simulink model "model_affc"  (R2016b)
settings: Solver=FixedStepDiscrete  StartTime=0.0  StopTime=inf  FixedStep=sampleTime  RelTol=1e-3
InitFcn:
  | model_affc_parameters;
StartFcn:
  | model_affc_parameters;
values from neighbouring files (symbols this model uses):
  Lb = 0.07    [model_affc_parameters.m]
  Lf = 0.238    [model_affc_parameters.m]
  Lu = 0.153    [model_affc_parameters.m]
  sampleTime = 0.001    [model_affc_parameters.m]
undefined symbols (not defined in the file or in its folder): FM1
libraries: simulink x11, LibraryFM x10, VariousBlocksLibrary x2, FMLibrary_v2 x1
settings Model: SimulationMode=external  Creator=niekbeckers  LastModifiedBy=Labuser
settings DataIOCC: LimitDataPoints=on  SaveFormat=Array
settings OptimizationCC: BlockReduction=off  BooleanDataType=off  LocalBlockOutputs=off  LifeSpan=inf
settings DebuggingCC: SaveWithParameterizedLinksMsg=none  UnderspecifiedInitializationDetection=Classic  MergeDetectMultiDrivingBlocksExec=none  SignalResolutionControl=TryResolveAllWithWarning  SFUnexpectedBacktrackingDiag=warning  SFNoUnconditionalDefaultTransitionDiag=warning  SFExecutionAtInitializationDiag=none
settings HardwareCC: ProdBitPerPointer=32  ProdBitPerSizeT=32  ProdBitPerPtrDiffT=32  ProdLargestAtomicFloat=None  ProdIntDivRoundTo=Undefined  ProdEndianess=Unspecified  ProdWordSize=32  ProdHWDeviceType=32-bit Generic  TargetBitPerPointer=64  TargetBitPerSizeT=64  TargetBitPerPtrDiffT=64  TargetLongLongMode=on  TargetIntDivRoundTo=Zero  TargetEndianess=LittleEndian  TargetWordSize=64  TargetHWDeviceType=MATLAB Host  ProdEqTarget=off
settings ModelReferenceCC: PropagateSignalLabelsOutOfModel=off
settings RTWCC: SystemTargetFile=TwinCAT.tlc  GenCodeOnly=on  MakeCommand=make_tct  TemplateMakefile=tct_msbuild.tmf  Description=TwinCAT Target  GenerateReport=on  TargetLang=C++
settings STFCustomTargetCC: CompOptLevelCompliant=on  GeneratePreprocessorConditionals=Disable all  MATLABClassNameForMDSCustomization=Simulink.SoftwareTarget.TargetSpecificTriggerConfigurationBase  SystemTargetFile=TwinCAT.tlc
settings ConfigComp: CovMetricSettings=dw  CovHtmlReporting=on  CovSaveCumulativeToWorkspaceVar=on  CovSaveSingleToWorkspaceVar=on  CovExternalEMLEnable=off  CovSFcnEnable=off

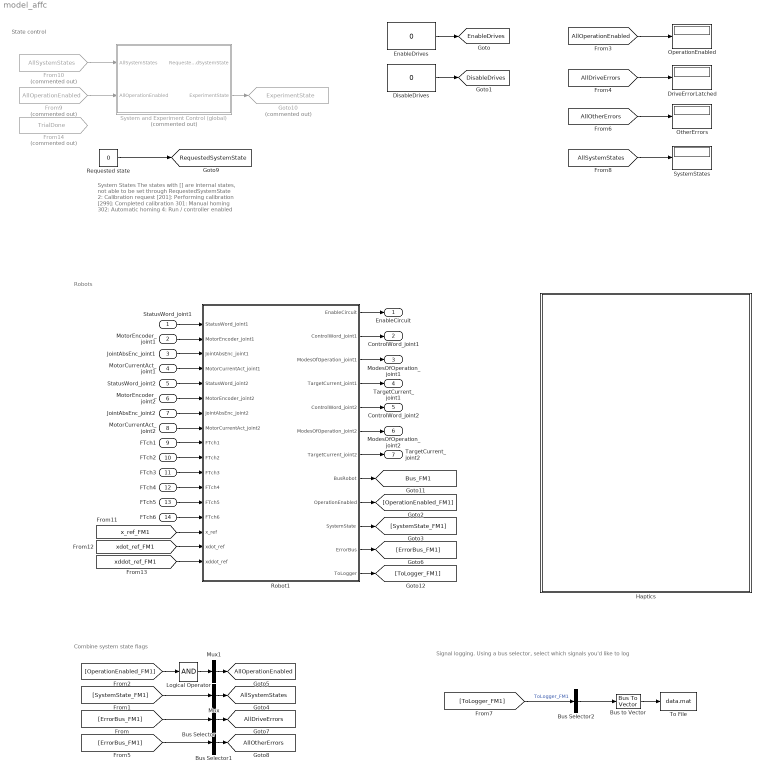
== system model_affc ==
  note: Signal logging.
      | Using a bus selector, select which signals you'd like to log
  note: System States
      | The states with [] are internal states, not able to be set through RequestedSystemState
      | 2: Calibration request
      | [201]: Performing calibration
      | [299]: Completed calibration
      | 301: Manual homing
      | 302: Automatic homing
      | 4: Run / controller enabled
  note: State control
  note: Combine system state flags
  note: Robots
  StatusWord_joint1 : Inport  OutDataTypeStr=uint16  PortDimensions=1
  MotorEncoder_joint1 : Inport  Port=2  OutDataTypeStr=int32  PortDimensions=1
  JointAbsEnc_joint1 : Inport  Port=3  OutDataTypeStr=int32  PortDimensions=1
  MotorCurrentAct_joint1 : Inport  Port=4  OutDataTypeStr=int16  PortDimensions=1
  StatusWord_joint2 : Inport  Port=5  OutDataTypeStr=uint16  PortDimensions=1
  MotorEncoder_joint2 : Inport  Port=6  OutDataTypeStr=int32  PortDimensions=1
  JointAbsEnc_joint2 : Inport  Port=7  OutDataTypeStr=int32  PortDimensions=1
  MotorCurrentAct_joint2 : Inport  Port=8  OutDataTypeStr=int16  PortDimensions=1
  FTch1 : Inport  Port=9  OutDataTypeStr=single  PortDimensions=1
  FTch2 : Inport  Port=10  OutDataTypeStr=single  PortDimensions=1
  FTch3 : Inport  Port=11  OutDataTypeStr=single  PortDimensions=1
  FTch4 : Inport  Port=12  OutDataTypeStr=single  PortDimensions=1
  FTch5 : Inport  Port=13  OutDataTypeStr=single  PortDimensions=1
  FTch6 : Inport  Port=14  OutDataTypeStr=single  PortDimensions=1
  Bus Selector : BusSelector  OutputSignals=DriveErrorLatched  OutputAsBus=on
  Bus Selector1 : BusSelector  OutputSignals=WorkspaceErrorLatched,ForceSensorLatched  OutputAsBus=on
  Bus Selector2 : BusSelector  OutputSignals=SystemState,ToLogger_ToEtherCAT.ToLogger_Actuator1.JointPosition_rad,ToLogger_ToEtherCAT.ToLogger_Actuator1.JointVelocity_rads,ToLogger_ToEtherCAT.ToLogger_Actuator1.JointTorque_Act_Nm,ToLogger_ToEtherCAT.ToLogger_Actuator1.DesiredTorqueLimited_Nm,ToLogger_ToEtherCAT.ToLogger_Actuator1.DriveError,ToLogger_ToEtherCAT.ToLogger_Actuator2.JointPosition_rad,ToLogger_ToEtherCAT.ToLogger_Actuator2.JointVelocity_rads,ToLogger_ToEtherCAT.ToLogger_Actuator2.JointTorque_Act_Nm,ToLogger_ToEtherCAT.ToLogger_Actuator2.DesiredTorqueLimited_Nm,ToLogger_ToEtherCAT.ToLogger_Actuator2.DriveError,ToLogger_Controller.q_ref,ToLogger_Controller.qdot_ref,ToLogger_Controller.qddot_ref  OutputAsBus=on
  Bus to Vector : BusToVector
  DisableDrives : Constant  Value=0
      settings: OpenFcn=set_param(gcb,'Value','1');tname = ['toggletimer_' gcb];delete(timerfind('name',tname));t = timer('timerfcn', ['set_param(''',gcb,''',''Value'',''0'')'],'executionmode','singleshot','startdelay',1,'name',tname);start(t);
      mask Display: fprintf('PushToTrigger\n%s',get_param(gcb,'value'))
  DriveErrorLatched : Display
  EnableDrives : Constant  Value=0
      settings: OpenFcn=set_param(gcb,'Value','1');tname = ['toggletimer_' gcb];delete(timerfind('name',tname));t = timer('timerfcn', ['set_param(''',gcb,''',''Value'',''0'')'],'executionmode','singleshot','startdelay',1,'name',tname);start(t);
      mask Display: fprintf('PushToTrigger\n%s',get_param(gcb,'value'))
  From10 : From  Commented=on  GotoTag=AllSystemStates
  From14 : From  Commented=on  GotoTag=TrialDone
  From9 : From  Commented=on  GotoTag=AllOperationEnabled
  Goto10 : Goto  Commented=on  GotoTag=ExperimentState  TagVisibility=global
  Haptics : Subsystem
  Logical Operator : Logic  Inputs=1  AllPortsSameDT=off  OutDataTypeStr=boolean
  Mux : Mux  Inputs=1
  Mux1 : Mux  Inputs=1
  OperationEnabled : Display
  OtherErrors : Display
  Requested state : Constant  Value=0
  Robot1 : Subsystem  AncestorBlock=LibraryFM/Robot1  mask{RobotStruct=FM1}
      mask prompts: RobotStruct "Robot struct (data)"
  System and Experiment Control (global) : Subsystem  Commented=on
  SystemStates : Display
  To File : ToFile  Filename=data.mat
  EnableCircuit : Outport  OutDataTypeStr=boolean  PortDimensions=1
  ControlWord_joint1 : Outport  Port=2  OutDataTypeStr=uint16  PortDimensions=1
  ModesOfOperation_joint1 : Outport  Port=3  OutDataTypeStr=int8  PortDimensions=1
  TargetCurrent_joint1 : Outport  Port=4  OutDataTypeStr=int16  PortDimensions=1
  ControlWord_joint2 : Outport  Port=5  OutDataTypeStr=uint16  PortDimensions=1
  ModesOfOperation_joint2 : Outport  Port=6  OutDataTypeStr=int8  PortDimensions=1
  TargetCurrent_joint2 : Outport  Port=7  OutDataTypeStr=int16  PortDimensions=1
  tag scope: AllDriveErrors=global, AllOperationEnabled=global, AllOtherErrors=global, AllSystemStates=global, Bus_FM1=global, DisableDrives=global, EnableDrives=global, RequestedSystemState=global
  wires:
  DisableDrives/1 -> [DisableDrives]
  EnableDrives/1 -> [EnableDrives]
  Robot1/9(OperationEnabled) -> [OperationEnabled_FM1]
  [AllOperationEnabled] -> OperationEnabled/1
  Robot1/10(SystemState) -> [SystemState_FM1]
  [SystemState_FM1] -> Mux/1
  Mux/1 -> [AllSystemStates]
  Mux1/1 -> [AllOperationEnabled]
  [OperationEnabled_FM1] -> Logical Operator/1
  Robot1/11(ErrorBus) -> [ErrorBus_FM1]
  [ErrorBus_FM1] -> Bus Selector/1
  Bus Selector/1 -> [AllDriveErrors]
  [AllDriveErrors] -> DriveErrorLatched/1
  [ErrorBus_FM1] -> Bus Selector1/1
  Bus Selector1/1 -> [AllOtherErrors]
  [AllOtherErrors] -> OtherErrors/1
  [AllSystemStates] -> SystemStates/1
  System and Experiment Control (global)/2(ExperimentState) -> Goto10/1
  From10/1 -> System and Experiment Control (global)/1(AllSystemStates)
  From9/1 -> System and Experiment Control (global)/2(AllOperationEnabled)
  [x_ref_FM1] -> Robot1/15(x_ref)
  [xdot_ref_FM1] -> Robot1/16(xdot_ref)
  [xddot_ref_FM1] -> Robot1/17(xddot_ref)
  Requested state/1 -> [RequestedSystemState]
  Robot1/8(BusRobot) -> [Bus_FM1]
  StatusWord_joint1/1 -> Robot1/1(StatusWord_joint1)
  MotorEncoder_joint1/1 -> Robot1/2(MotorEncoder_joint1)
  JointAbsEnc_joint1/1 -> Robot1/3(JointAbsEnc_joint1)
  MotorCurrentAct_joint1/1 -> Robot1/4(MotorCurrentAct_joint1)
  StatusWord_joint2/1 -> Robot1/5(StatusWord_joint2)
  MotorEncoder_joint2/1 -> Robot1/6(MotorEncoder_joint2)
  JointAbsEnc_joint2/1 -> Robot1/7(JointAbsEnc_joint2)
  MotorCurrentAct_joint2/1 -> Robot1/8(MotorCurrentAct_joint2)
  FTch1/1 -> Robot1/9(FTch1)
  FTch2/1 -> Robot1/10(FTch2)
  FTch3/1 -> Robot1/11(FTch3)
  FTch4/1 -> Robot1/12(FTch4)
  FTch5/1 -> Robot1/13(FTch5)
  FTch6/1 -> Robot1/14(FTch6)
  Robot1/1(EnableCircuit) -> EnableCircuit/1
  Robot1/2(ControlWord_joint1) -> ControlWord_joint1/1
  Robot1/3(ModesOfOperation_joint1) -> ModesOfOperation_joint1/1
  Robot1/4(TargetCurrent_joint1) -> TargetCurrent_joint1/1
  Robot1/7(TargetCurrent_joint2) -> TargetCurrent_joint2/1
  Robot1/6(ModesOfOperation_joint2) -> ModesOfOperation_joint2/1
  Robot1/5(ControlWord_joint2) -> ControlWord_joint2/1
  Robot1/12(ToLogger) -> [ToLogger_FM1]
  [ToLogger_FM1] -> Bus Selector2/1  "ToLogger_FM1"
  Bus Selector2/1 -> Bus to Vector/1
  Bus to Vector/1 -> To File/1
  Logical Operator/1 -> Mux1/1

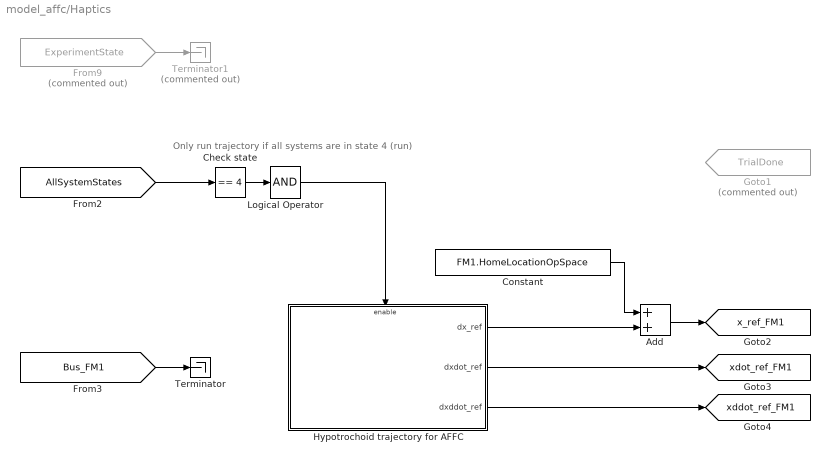
== system model_affc/Haptics ==
  note: Only run trajectory if all systems are in state 4 (run)
  Add : Sum
  "Check state " : simulink/Logic and Bit Operations/Compare To Constant  relop===  const=4  OutDataTypeStr=boolean
  Constant : Constant  Value=FM1.HomeLocationOpSpace
  From9 : From  Commented=on  GotoTag=ExperimentState
  Goto1 : Goto  Commented=on  GotoTag=TrialDone  TagVisibility=global
  Hypotrochoid trajectory for AFFC : Subsystem
  Logical Operator : Logic  Inputs=1  AllPortsSameDT=off  OutDataTypeStr=boolean
  Terminator : Terminator
  Terminator1 : Terminator  Commented=on
  tag scope: x_ref_FM1=global, xddot_ref_FM1=global, xdot_ref_FM1=global
  wires:
  [Bus_FM1] -> Terminator/1
  Constant/1 -> Add/1
  Hypotrochoid trajectory for AFFC/1(dx_ref) -> Add/2
  Add/1 -> [x_ref_FM1]
  Hypotrochoid trajectory for AFFC/2(dxdot_ref) -> [xdot_ref_FM1]
  Hypotrochoid trajectory for AFFC/3(dxddot_ref) -> [xddot_ref_FM1]
  [AllSystemStates] -> "Check state "/1
  "Check state "/1 -> Logical Operator/1
  Logical Operator/1 -> Hypotrochoid trajectory for AFFC/Enable
  From9/1 -> Terminator1/1

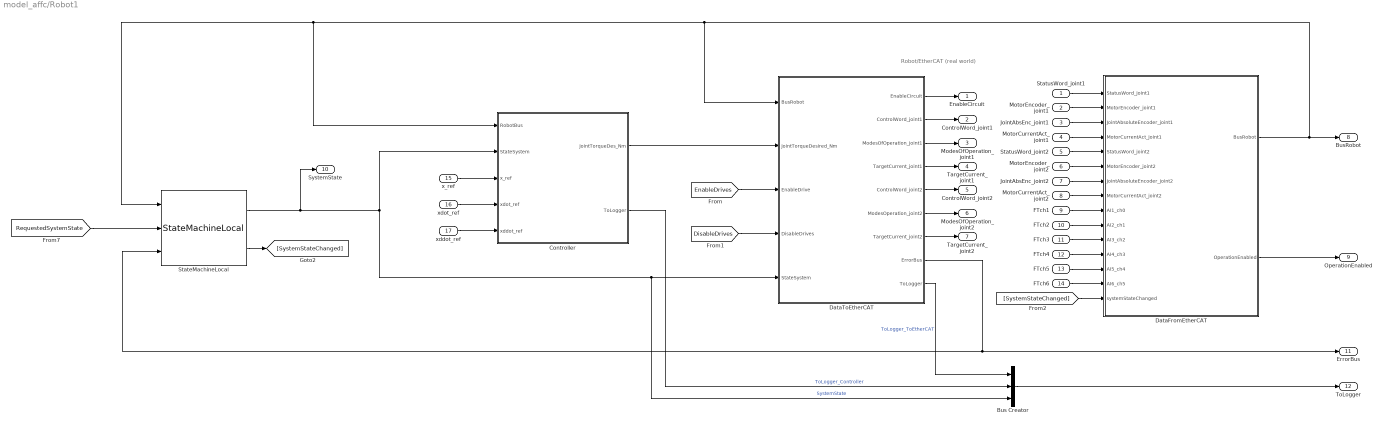
== system model_affc/Robot1 ==
  note: Robot/EtherCAT (real world)
  StatusWord_joint1 : Inport
  MotorEncoder_joint1 : Inport  Port=2
  JointAbsEnc_joint1 : Inport  Port=3
  MotorCurrentAct_joint1 : Inport  Port=4
  StatusWord_joint2 : Inport  Port=5
  MotorEncoder_joint2 : Inport  Port=6
  JointAbsEnc_joint2 : Inport  Port=7
  MotorCurrentAct_joint2 : Inport  Port=8
  FTch1 : Inport  Port=9
  FTch2 : Inport  Port=10
  FTch3 : Inport  Port=11
  FTch4 : Inport  Port=12
  FTch5 : Inport  Port=13
  FTch6 : Inport  Port=14
  x_ref : Inport  Port=15
  xdot_ref : Inport  Port=16
  xddot_ref : Inport  Port=17
  Bus Creator : BusCreator  Inputs=3
  Controller : Subsystem  AncestorBlock=LibraryFM/Controller
  DataFromEtherCAT : Subsystem  AncestorBlock=LibraryFM/DataFromEtherCAT
  DataToEtherCAT : Subsystem  AncestorBlock=LibraryFM/DataToEtherCAT
  StateMachineLocal : LibraryFM/StateMachineLocal
  EnableCircuit : Outport
  ControlWord_joint1 : Outport  Port=2
  ModesOfOperation_joint1 : Outport  Port=3
  TargetCurrent_joint1 : Outport  Port=4
  ControlWord_joint2 : Outport  Port=5
  ModesOfOperation_joint2 : Outport  Port=6
  TargetCurrent_joint2 : Outport  Port=7
  BusRobot : Outport  Port=8
  OperationEnabled : Outport  Port=9
  SystemState : Outport  Port=10
  ErrorBus : Outport  Port=11
  ToLogger : Outport  Port=12
  wires:
  Controller/2(ToLogger) -> Bus Creator/2  "ToLogger_Controller"
  DataToEtherCAT/9(ToLogger) -> Bus Creator/1  "ToLogger_ToEtherCAT"
  Bus Creator/1 -> ToLogger/1
  xddot_ref/1 -> Controller/5(xddot_ref)
  xdot_ref/1 -> Controller/4(xdot_ref)
  x_ref/1 -> Controller/3(x_ref)
  DataToEtherCAT/7(TargetCurrent_joint2) -> TargetCurrent_joint2/1
  FTch2/1 -> DataFromEtherCAT/10(AI2_ch1)
  MotorCurrentAct_joint1/1 -> DataFromEtherCAT/4(MotorCurrentAct_joint1)
  MotorEncoder_joint2/1 -> DataFromEtherCAT/6(MotorEncoder_joint2)
  JointAbsEnc_joint1/1 -> DataFromEtherCAT/3(JointAbsoluteEncoder_joint1)
  DataToEtherCAT/3(ModesOfOperation_joint1) -> ModesOfOperation_joint1/1
  DataToEtherCAT/1(EnableCircuit) -> EnableCircuit/1
  FTch1/1 -> DataFromEtherCAT/9(AI1_ch0)
  StateMachineLocal/1 -> Bus Creator/3, DataToEtherCAT/5(StateSystem), Controller/2(StateSystem), SystemState/1  "SystemState"
  DataToEtherCAT/2(ControlWord_joint1) -> ControlWord_joint1/1
  StateMachineLocal/2 -> [SystemStateChanged]
  [SystemStateChanged] -> DataFromEtherCAT/15(systemStateChanged)
  DataToEtherCAT/8(ErrorBus) -> ErrorBus/1, StateMachineLocal/3
  DataFromEtherCAT/1(BusRobot) -> StateMachineLocal/1, Controller/1(RobotBus), DataToEtherCAT/1(BusRobot), BusRobot/1
  [RequestedSystemState] -> StateMachineLocal/2
  Controller/1(JointTorqueDes_Nm) -> DataToEtherCAT/2(JointTorqueDesired_Nm)
  [DisableDrives] -> DataToEtherCAT/4(DisableDrives)
  [EnableDrives] -> DataToEtherCAT/3(EnableDrive)
  MotorCurrentAct_joint2/1 -> DataFromEtherCAT/8(MotorCurrentAct_joint2)
  DataToEtherCAT/4(TargetCurrent_joint1) -> TargetCurrent_joint1/1
  FTch5/1 -> DataFromEtherCAT/13(AI5_ch4)
  JointAbsEnc_joint2/1 -> DataFromEtherCAT/7("JointAbsoluteEncoder_joint2 ")
  MotorEncoder_joint1/1 -> DataFromEtherCAT/2(MotorEncoder_joint1)
  DataToEtherCAT/5(ControlWord_joint2) -> ControlWord_joint2/1
  DataToEtherCAT/6(ModesOperation_joint2) -> ModesOfOperation_joint2/1
  StatusWord_joint1/1 -> DataFromEtherCAT/1(StatusWord_joint1)
  StatusWord_joint2/1 -> DataFromEtherCAT/5(StatusWord_joint2)
  FTch6/1 -> DataFromEtherCAT/14(AI6_ch5)
  FTch4/1 -> DataFromEtherCAT/12(AI4_ch3)
  FTch3/1 -> DataFromEtherCAT/11(AI3_ch2)
  DataFromEtherCAT/2(OperationEnabled) -> OperationEnabled/1

== system model_affc/System and Experiment Control (global) ==
  note: Hier ergens experiment protocol inlezen
  AllSystemStates : Inport
  AllOperationEnabled : Inport  Port=2
  GlobalStateMachine : FMLibrary_v2/StateMachineLocal/SystemLocalStateMachine
  RequestedSystemState : Outport
  ExperimentState : Outport  Port=2
  wires:
  GlobalStateMachine/1 -> RequestedSystemState/1

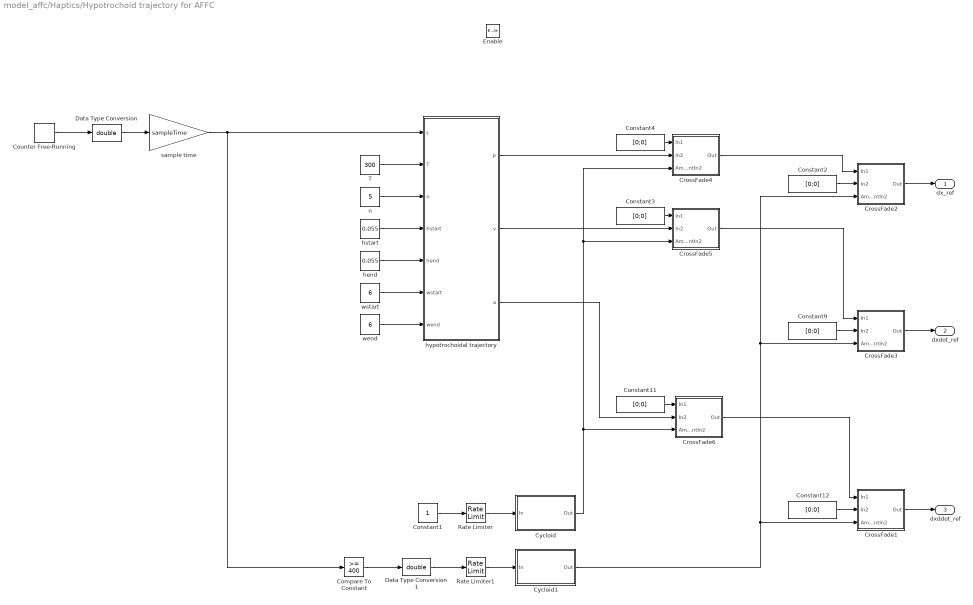
== system model_affc/Haptics/Hypotrochoid trajectory for AFFC ==
  Enable : EnablePort  StatesWhenEnabling=reset
  Compare To Constant : simulink/Logic and Bit Operations/Compare To Constant  relop=>=  const=400  OutDataTypeStr=boolean
  Constant1 : Constant
  Constant{2..4,9,11..12} (6 alike) : Constant  Value=[0;0]
  Counter Free-Running : simulink/Sources/Counter Free-Running  NumBits=32  tsamp=-1
  CrossFade1 : Subsystem  AncestorBlock=VariousBlocksLibrary/Various/CrossFade
  CrossFade2 : Subsystem  AncestorBlock=VariousBlocksLibrary/Various/CrossFade
  CrossFade3 : Subsystem  AncestorBlock=VariousBlocksLibrary/Various/CrossFade
  CrossFade4 : Subsystem
  CrossFade5 : Subsystem  AncestorBlock=VariousBlocksLibrary/Various/CrossFade
  CrossFade6 : Subsystem  AncestorBlock=VariousBlocksLibrary/Various/CrossFade
  Cycloid : Subsystem  AncestorBlock=VariousBlocksLibrary/Various/Cycloid
  Cycloid1 : Subsystem  AncestorBlock=VariousBlocksLibrary/Various/Cycloid
  Data Type Conversion : DataTypeConversion  OutDataTypeStr=double
  Data Type Conversion1 : DataTypeConversion  OutDataTypeStr=double
  Rate Limiter : RateLimiter  RisingSlewLimit=0.25  FallingSlewLimit=-0.15  SampleTimeMode=inherited
  Rate Limiter1 : RateLimiter  RisingSlewLimit=0.2  FallingSlewLimit=-0.2  SampleTimeMode=inherited
  T : Constant  Value=300
  hend : Constant  Value=0.055
  hstart : Constant  Value=0.055
  hypotrochoidal trajectory : MATLAB Function  TreatAsAtomicUnit=on
  n : Constant  Value=5
  sample time : Gain  Gain=sampleTime
  wend : Constant  Value=6
  wstart : Constant  Value=6
  dx_ref : Outport
  dxdot_ref : Outport  Port=2
  dxddot_ref : Outport  Port=3
  wires:
  Data Type Conversion1/1 -> Rate Limiter1/1
  hypotrochoidal trajectory/1(p) -> CrossFade4/2(In2)
  CrossFade1/1(Out) -> dxddot_ref/1
  Constant11/1 -> CrossFade6/1(In1)
  Constant12/1 -> CrossFade1/2(In2)
  CrossFade6/1(Out) -> CrossFade1/1(In1)
  Constant9/1 -> CrossFade3/2(In2)
  CrossFade5/1(Out) -> CrossFade3/1(In1)
  CrossFade3/1(Out) -> dxdot_ref/1
  Cycloid1/1(Out) -> CrossFade1/3(AmountIn2), CrossFade2/3(AmountIn2), CrossFade3/3(AmountIn2)
  Rate Limiter1/1 -> Cycloid1/1(In)
  Compare To Constant/1 -> Data Type Conversion1/1
  CrossFade4/1(Out) -> CrossFade2/1(In1)
  CrossFade2/1(Out) -> dx_ref/1
  Rate Limiter/1 -> Cycloid/1(In)
  Constant1/1 -> Rate Limiter/1
  Cycloid/1(Out) -> CrossFade6/3(AmountIn2), CrossFade5/3(AmountIn2), CrossFade4/3(AmountIn2)
  hypotrochoidal trajectory/2(v) -> CrossFade5/2(In2)
  hypotrochoidal trajectory/3(a) -> CrossFade6/2(In2)
  sample time/1 -> Compare To Constant/1, hypotrochoidal trajectory/1(t)
  Constant2/1 -> CrossFade2/2(In2)
  Data Type Conversion/1 -> sample time/1
  wstart/1 -> hypotrochoidal trajectory/6(wstart)
  wend/1 -> hypotrochoidal trajectory/7(wend)
  hstart/1 -> hypotrochoidal trajectory/4(hstart)
  hend/1 -> hypotrochoidal trajectory/5(hend)
  n/1 -> hypotrochoidal trajectory/3(n)
  T/1 -> hypotrochoidal trajectory/2(T)
  Counter Free-Running/1 -> Data Type Conversion/1
  Constant3/1 -> CrossFade5/1(In1)
  Constant4/1 -> CrossFade4/1(In1)

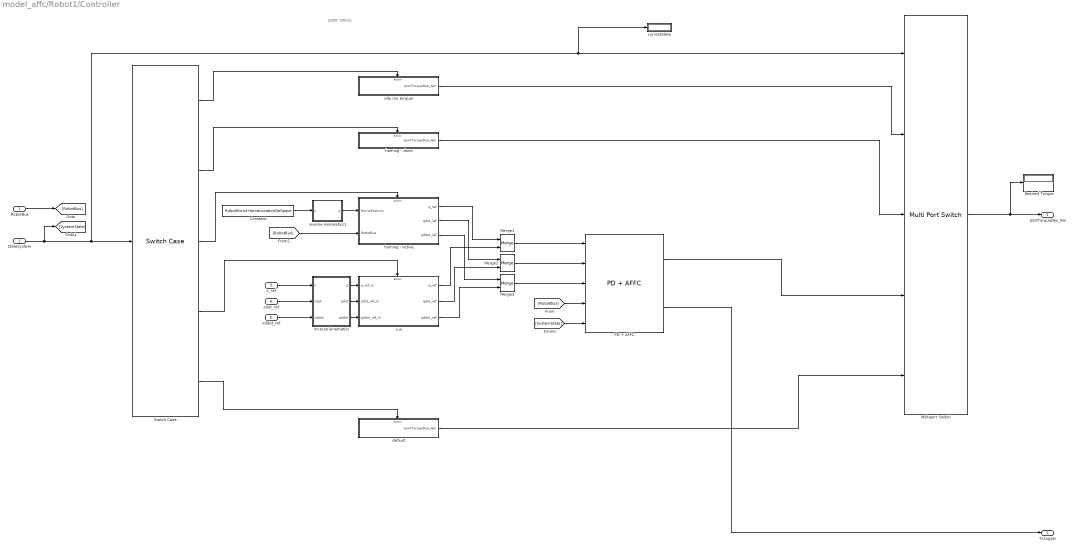
== system model_affc/Robot1/Controller ==
  note: JOINT SPACE
  RobotBus : Inport
  StateSystem : Inport  Port=2
  x_ref : Inport  Port=3
  xdot_ref : Inport  Port=4
  xddot_ref : Inport  Port=5
  Constant : Constant  Value=RobotStruct.HomeLocationOpSpace
  Desired Torque : Display
  Merge1 : Merge
  Merge2 : Merge
  Merge3 : Merge
  Multiport Switch : MultiPortSwitch  DataPortOrder=Specify indices  Inputs=4  DataPortIndices={[0,1,2,201,299,301],[399],[302,4]}  DataPortForDefault=Additional data port
  PD + AFFC : LibraryFM/PD + AFFC
      link override AFFC/p: InitialOutput=zeros(7,1)
  Switch Case : SwitchCase  CaseConditions={[0,1,2,201,299,301],[399],[302],[4]}
  currentState : Display
  default : Subsystem  TreatAsAtomicUnit=on
  homing - active : Subsystem
  homing - done : Subsystem  TreatAsAtomicUnit=on
  idle (no torque) : Subsystem  TreatAsAtomicUnit=on
  inverse kinematics : MATLAB Function  TreatAsAtomicUnit=on
  inverse kinematics1 : MATLAB Function  TreatAsAtomicUnit=on
  run : Subsystem
  JointTorqueDes_Nm : Outport
  ToLogger : Outport  Port=2
  wires:
  PD + AFFC/2 -> ToLogger/1
  xdot_ref/1 -> inverse kinematics/2(xdot)
  xddot_ref/1 -> inverse kinematics/3(xddot)
  x_ref/1 -> inverse kinematics/1(x)
  [SystemState] -> PD + AFFC/5
  inverse kinematics1/1(q) -> homing - active/1(HomePosition)
  inverse kinematics/3(qddot) -> run/3(qddot_ref_in)
  inverse kinematics/2(qdot) -> run/2(qdot_ref_in)
  inverse kinematics/1(q) -> run/1(q_ref_in)
  Constant/1 -> inverse kinematics1/1(x)
  [RobotBus] -> homing - active/2(RobotBus)
  [RobotBus] -> PD + AFFC/4
  RobotBus/1 -> [RobotBus]
  PD + AFFC/1 -> Multiport Switch/4
  Merge3/1 -> PD + AFFC/3
  Merge2/1 -> PD + AFFC/2
  Merge1/1 -> PD + AFFC/1
  homing - done/1(JointTorqueDes_Nm) -> Multiport Switch/3
  idle (no torque)/1(JointTorqueDes_Nm) -> Multiport Switch/2
  Switch Case/2 -> homing - done/Action
  Switch Case/3 -> homing - active/Action
  Switch Case/1 -> idle (no torque)/Action
  default/1(JointTorqueDes_Nm) -> Multiport Switch/5
  Switch Case/5 -> default/Action
  Multiport Switch/1 -> Desired Torque/1, JointTorqueDes_Nm/1
  Switch Case/4 -> run/Action
  homing - active/1(q_ref) -> Merge1/1
  run/1(q_ref) -> Merge1/2
  StateSystem/1 -> Multiport Switch/1, currentState/1, Switch Case/1, [SystemState]
  run/2(qdot_ref) -> Merge2/2
  run/3(qddot_ref) -> Merge3/2
  homing - active/2(qdot_ref) -> Merge2/1
  homing - active/3(qddot_ref) -> Merge3/1

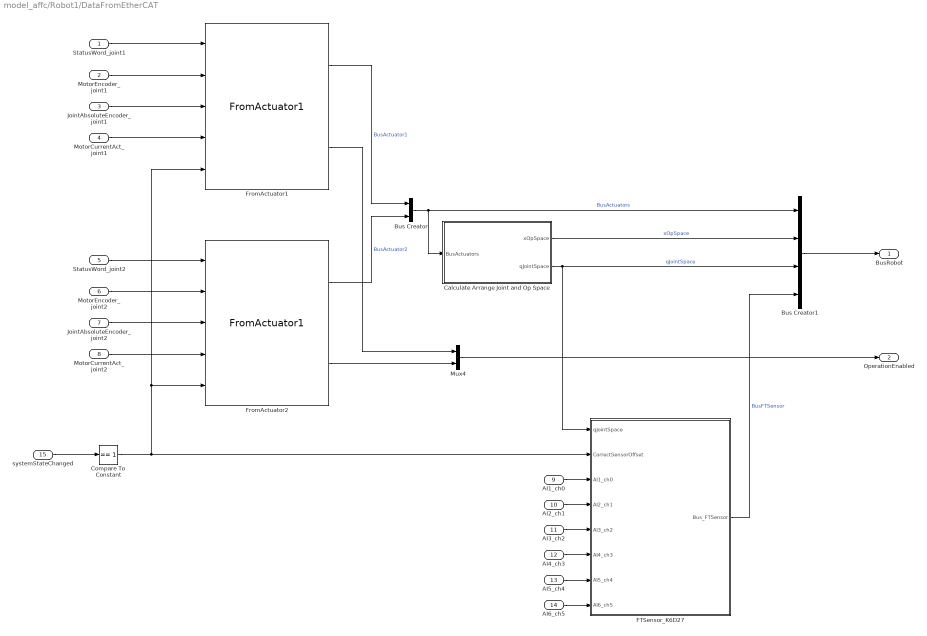
== system model_affc/Robot1/DataFromEtherCAT ==
  StatusWord_joint1 : Inport
  MotorEncoder_joint1 : Inport  Port=2
  JointAbsoluteEncoder_joint1 : Inport  Port=3
  MotorCurrentAct_joint1 : Inport  Port=4
  StatusWord_joint2 : Inport  Port=5
  MotorEncoder_joint2 : Inport  Port=6
  "JointAbsoluteEncoder_joint2 " : Inport  Port=7
  MotorCurrentAct_joint2 : Inport  Port=8
  AI1_ch0 : Inport  Port=9
  AI2_ch1 : Inport  Port=10
  AI3_ch2 : Inport  Port=11
  AI4_ch3 : Inport  Port=12
  AI5_ch4 : Inport  Port=13
  AI6_ch5 : Inport  Port=14
  systemStateChanged : Inport  Port=15
  Bus Creator : BusCreator  Inputs=2
  Bus Creator1 : BusCreator  Inputs=4
  Calculate Arrange Joint and Op Space : Subsystem
  Compare To Constant : simulink/Logic and Bit Operations/Compare To Constant  relop===  const=1  OutDataTypeStr=boolean
  FTSensor_K6D27 : Subsystem  mask{FTSensorStruct=RobotStruct.FTSensor}
      mask prompts: FTSensorStruct "Struct for force torque sensor"
  FromActuator1 : LibraryFM/FromActuator1  ActuatorStruct=RobotStruct.Actuator1
  FromActuator2 : LibraryFM/FromActuator1  ActuatorStruct=RobotStruct.Actuator2
  Mux4 : Mux  Inputs=2
  BusRobot : Outport
  OperationEnabled : Outport  Port=2
  wires:
  FromActuator1/1 -> Bus Creator/1  "BusActuator1"
  FromActuator2/1 -> Bus Creator/2  "BusActuator2"
  FromActuator1/2 -> Mux4/1
  Mux4/1 -> OperationEnabled/1
  FromActuator2/2 -> Mux4/2
  MotorEncoder_joint1/1 -> FromActuator1/2
  StatusWord_joint1/1 -> FromActuator1/1
  JointAbsoluteEncoder_joint1/1 -> FromActuator1/3
  MotorCurrentAct_joint1/1 -> FromActuator1/4
  MotorEncoder_joint2/1 -> FromActuator2/2
  StatusWord_joint2/1 -> FromActuator2/1
  "JointAbsoluteEncoder_joint2 "/1 -> FromActuator2/3
  MotorCurrentAct_joint2/1 -> FromActuator2/4
  Bus Creator/1 -> Calculate Arrange Joint and Op Space/1(BusActuators), Bus Creator1/1  "BusActuators"
  Bus Creator1/1 -> BusRobot/1
  Calculate Arrange Joint and Op Space/1(xOpSpace) -> Bus Creator1/2  "xOpSpace"
  Calculate Arrange Joint and Op Space/2(qJointSpace) -> FTSensor_K6D27/1(qJointSpace), Bus Creator1/3  "qJointSpace"
  systemStateChanged/1 -> Compare To Constant/1
  AI1_ch0/1 -> FTSensor_K6D27/3(AI1_ch0)
  AI2_ch1/1 -> FTSensor_K6D27/4(AI2_ch1)
  AI3_ch2/1 -> FTSensor_K6D27/5(AI3_ch2)
  AI4_ch3/1 -> FTSensor_K6D27/6(AI4_ch3)
  AI5_ch4/1 -> FTSensor_K6D27/7(AI5_ch4)
  AI6_ch5/1 -> FTSensor_K6D27/8(AI6_ch5)
  Compare To Constant/1 -> FromActuator1/5, FromActuator2/5, FTSensor_K6D27/2(CorrectSensorOffset)
  FTSensor_K6D27/1(Bus_FTSensor) -> Bus Creator1/4  "BusFTSensor"

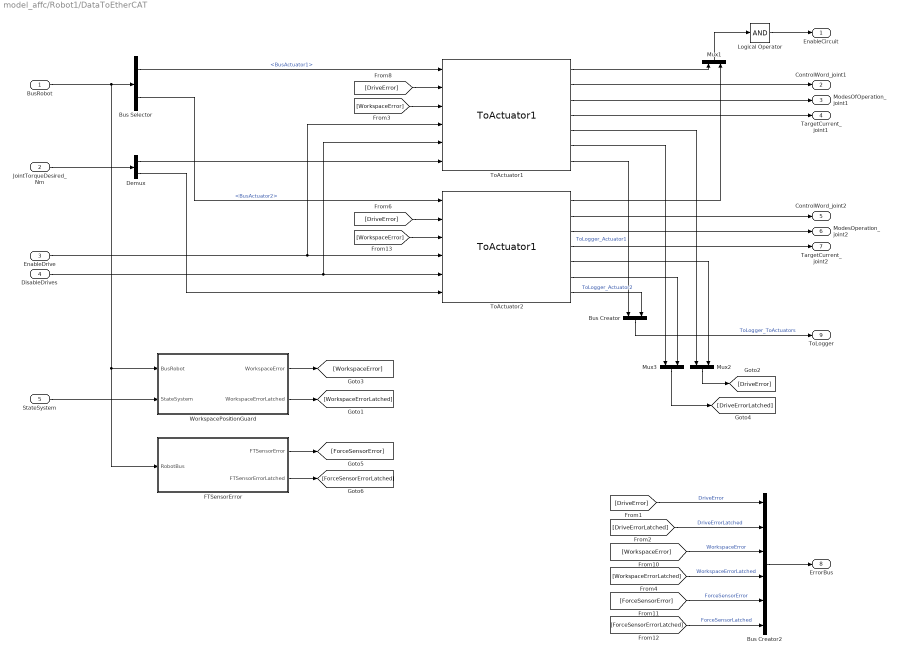
== system model_affc/Robot1/DataToEtherCAT ==
  BusRobot : Inport
  JointTorqueDesired_Nm : Inport  Port=2
  EnableDrive : Inport  Port=3
  DisableDrives : Inport  Port=4
  StateSystem : Inport  Port=5
  Bus Creator : BusCreator  Inputs=2
  Bus Creator2 : BusCreator  Inputs=6
  Bus Selector : BusSelector  OutputSignals=BusActuators.BusActuator1,BusActuators.BusActuator2
  Demux : Demux  Outputs=2
  FTSensorError : Subsystem
  Logical Operator : Logic  Inputs=1  AllPortsSameDT=off  OutDataTypeStr=boolean
  Mux1 : Mux  Inputs=2
  Mux2 : Mux  Inputs=2
  Mux3 : Mux  Inputs=2
  ToActuator1 : LibraryFM/ToActuator1  ActuatorStruct=RobotStruct.Actuator1
  ToActuator2 : LibraryFM/ToActuator1  ActuatorStruct=RobotStruct.Actuator2
  WorkspacePositionGuard : Subsystem
  EnableCircuit : Outport  OutDataTypeStr=boolean
  ControlWord_joint1 : Outport  Port=2  OutDataTypeStr=uint16
  ModesOfOperation_joint1 : Outport  Port=3  OutDataTypeStr=int8
  TargetCurrent_joint1 : Outport  Port=4  OutDataTypeStr=int16
  ControlWord_joint2 : Outport  Port=5  OutDataTypeStr=uint16
  ModesOperation_joint2 : Outport  Port=6  OutDataTypeStr=int8
  TargetCurrent_joint2 : Outport  Port=7  OutDataTypeStr=int16
  ErrorBus : Outport  Port=8
  ToLogger : Outport  Port=9
  wires:
  Bus Creator/1 -> ToLogger/1  "ToLogger_ToActuators"
  ToActuator2/7 -> Bus Creator/2  "ToLogger_Actuator2"
  ToActuator1/7 -> Bus Creator/1  "ToLogger_Actuator1"
  ToActuator1/5 -> Mux2/1
  ToActuator2/5 -> Mux2/2
  Mux2/1 -> [DriveError]
  ToActuator1/6 -> Mux3/1
  ToActuator2/6 -> Mux3/2
  [DriveError] -> ToActuator1/2
  Mux1/1 -> Logical Operator/1
  ToActuator1/1 -> Mux1/1
  ToActuator2/1 -> Mux1/2
  ToActuator1/2 -> ControlWord_joint1/1
  ToActuator1/3 -> ModesOfOperation_joint1/1
  ToActuator2/2 -> ControlWord_joint2/1
  ToActuator1/4 -> TargetCurrent_joint1/1
  ToActuator2/4 -> TargetCurrent_joint2/1
  ToActuator2/3 -> ModesOperation_joint2/1
  Logical Operator/1 -> EnableCircuit/1
  Demux/2 -> ToActuator2/6
  JointTorqueDesired_Nm/1 -> Demux/1
  Demux/1 -> ToActuator1/6
  BusRobot/1 -> FTSensorError/1(RobotBus), WorkspacePositionGuard/1(BusRobot), Bus Selector/1
  Bus Selector/2 -> ToActuator2/1  "<BusActuator2>"
  Bus Selector/1 -> ToActuator1/1  "<BusActuator1>"
  WorkspacePositionGuard/2(WorkspaceErrorLatched) -> [WorkspaceErrorLatched]
  WorkspacePositionGuard/1(WorkspaceError) -> [WorkspaceError]
  [WorkspaceError] -> ToActuator1/3
  DisableDrives/1 -> ToActuator1/5, ToActuator2/5
  EnableDrive/1 -> ToActuator1/4, ToActuator2/4
  [DriveError] -> ToActuator2/2
  [WorkspaceError] -> ToActuator2/3
  Mux3/1 -> [DriveErrorLatched]
  Bus Creator2/1 -> ErrorBus/1
  [DriveError] -> Bus Creator2/1  "DriveError"
  [DriveErrorLatched] -> Bus Creator2/2  "DriveErrorLatched"
  [WorkspaceError] -> Bus Creator2/3  "WorkspaceError"
  [WorkspaceErrorLatched] -> Bus Creator2/4  "WorkspaceErrorLatched"
  StateSystem/1 -> WorkspacePositionGuard/2(StateSystem)
  FTSensorError/1(FTSensorError) -> [ForceSensorError]
  FTSensorError/2(FTSensorErrorLatched) -> [ForceSensorErrorLatched]
  [ForceSensorError] -> Bus Creator2/5  "ForceSensorError"
  [ForceSensorErrorLatched] -> Bus Creator2/6  "ForceSensorLatched"

== system model_affc/Haptics/Hypotrochoid trajectory for AFFC/CrossFade1 ==
  In1 : Inport
  In2 : Inport  Port=2
  AmountIn2 : Inport  Port=3
  Add : Sum  Inputs=+-
  Add1 : Sum
  One : Constant
  Product : Product  RndMeth=Zero
  Product1 : Product  RndMeth=Zero
  Saturation : Saturate  UpperLimit=1  LowerLimit=0
  Out : Outport
  wires:
  In1/1 -> Product1/1
  AmountIn2/1 -> Saturation/1
  One/1 -> Add/1
  Saturation/1 -> Product/2, Add/2
  Add/1 -> Product1/2
  Product/1 -> Add1/2
  Product1/1 -> Add1/1
  In2/1 -> Product/1
  Add1/1 -> Out/1

== system model_affc/Haptics/Hypotrochoid trajectory for AFFC/CrossFade2 ==
  In1 : Inport
  In2 : Inport  Port=2
  AmountIn2 : Inport  Port=3
  Add : Sum  Inputs=+-
  Add1 : Sum
  One : Constant
  Product : Product  RndMeth=Zero
  Product1 : Product  RndMeth=Zero
  Saturation : Saturate  UpperLimit=1  LowerLimit=0
  Out : Outport
  wires:
  In1/1 -> Product1/1
  AmountIn2/1 -> Saturation/1
  One/1 -> Add/1
  Saturation/1 -> Product/2, Add/2
  Add/1 -> Product1/2
  Product/1 -> Add1/2
  Product1/1 -> Add1/1
  In2/1 -> Product/1
  Add1/1 -> Out/1

== system model_affc/Haptics/Hypotrochoid trajectory for AFFC/CrossFade3 ==
  In1 : Inport
  In2 : Inport  Port=2
  AmountIn2 : Inport  Port=3
  Add : Sum  Inputs=+-
  Add1 : Sum
  One : Constant
  Product : Product  RndMeth=Zero
  Product1 : Product  RndMeth=Zero
  Saturation : Saturate  UpperLimit=1  LowerLimit=0
  Out : Outport
  wires:
  In1/1 -> Product1/1
  AmountIn2/1 -> Saturation/1
  One/1 -> Add/1
  Saturation/1 -> Product/2, Add/2
  Add/1 -> Product1/2
  Product/1 -> Add1/2
  Product1/1 -> Add1/1
  In2/1 -> Product/1
  Add1/1 -> Out/1

== system model_affc/Haptics/Hypotrochoid trajectory for AFFC/CrossFade4 ==
  In1 : Inport
  In2 : Inport  Port=2
  AmountIn2 : Inport  Port=3
  Add : Sum  Inputs=+-
  Add1 : Sum
  One : Constant
  Product : Product  RndMeth=Zero
  Product1 : Product  RndMeth=Zero
  Saturation : Saturate  UpperLimit=1  LowerLimit=0
  Out : Outport
  wires:
  In1/1 -> Product1/1
  AmountIn2/1 -> Saturation/1
  One/1 -> Add/1
  Saturation/1 -> Product/2, Add/2
  Add/1 -> Product1/2
  Product/1 -> Add1/2
  Product1/1 -> Add1/1
  In2/1 -> Product/1
  Add1/1 -> Out/1

== system model_affc/Haptics/Hypotrochoid trajectory for AFFC/CrossFade5 ==
  In1 : Inport
  In2 : Inport  Port=2
  AmountIn2 : Inport  Port=3
  Add : Sum  Inputs=+-
  Add1 : Sum
  One : Constant
  Product : Product  RndMeth=Zero
  Product1 : Product  RndMeth=Zero
  Saturation : Saturate  UpperLimit=1  LowerLimit=0
  Out : Outport
  wires:
  In1/1 -> Product1/1
  AmountIn2/1 -> Saturation/1
  One/1 -> Add/1
  Saturation/1 -> Product/2, Add/2
  Add/1 -> Product1/2
  Product/1 -> Add1/2
  Product1/1 -> Add1/1
  In2/1 -> Product/1
  Add1/1 -> Out/1

== system model_affc/Haptics/Hypotrochoid trajectory for AFFC/CrossFade6 ==
  In1 : Inport
  In2 : Inport  Port=2
  AmountIn2 : Inport  Port=3
  Add : Sum  Inputs=+-
  Add1 : Sum
  One : Constant
  Product : Product  RndMeth=Zero
  Product1 : Product  RndMeth=Zero
  Saturation : Saturate  UpperLimit=1  LowerLimit=0
  Out : Outport
  wires:
  In1/1 -> Product1/1
  AmountIn2/1 -> Saturation/1
  One/1 -> Add/1
  Saturation/1 -> Product/2, Add/2
  Add/1 -> Product1/2
  Product/1 -> Add1/2
  Product1/1 -> Add1/1
  In2/1 -> Product/1
  Add1/1 -> Out/1

== system model_affc/Haptics/Hypotrochoid trajectory for AFFC/Cycloid ==
  note: Given a linear input 0<=in<=1, it gives a cycloid output 0<=out<=1.
      | If In is outside the 0..1 range, it is limited to 0 or 1.
  In : Inport
  Gain1 : Gain  Gain=2*pi
  Gain2 : Gain  Gain=1/(2*pi)
  Saturation : Saturate  UpperLimit=1  LowerLimit=0
  Subtract : Sum  Inputs=+-
  Trigonometric Function : Trigonometry
  Out : Outport
  wires:
  Gain1/1 -> Trigonometric Function/1
  Subtract/1 -> Out/1
  In/1 -> Saturation/1
  Saturation/1 -> Gain1/1, Subtract/1
  Trigonometric Function/1 -> Gain2/1
  Gain2/1 -> Subtract/2

== system model_affc/Haptics/Hypotrochoid trajectory for AFFC/Cycloid1 ==
  note: Given a linear input 0<=in<=1, it gives a cycloid output 0<=out<=1.
      | If In is outside the 0..1 range, it is limited to 0 or 1.
  In : Inport
  Gain1 : Gain  Gain=2*pi
  Gain2 : Gain  Gain=1/(2*pi)
  Saturation : Saturate  UpperLimit=1  LowerLimit=0
  Subtract : Sum  Inputs=+-
  Trigonometric Function : Trigonometry
  Out : Outport
  wires:
  Gain1/1 -> Trigonometric Function/1
  Subtract/1 -> Out/1
  In/1 -> Saturation/1
  Saturation/1 -> Gain1/1, Subtract/1
  Trigonometric Function/1 -> Gain2/1
  Gain2/1 -> Subtract/2

== system model_affc/Robot1/Controller/default ==
  Action Port : ActionPort  InitializeStates=reset  ActionType=default
  Constant3 : Constant  Value=[0;0]
  JointTorqueDes_Nm : Outport  InitialOutput=[0;0]
  wires:
  Constant3/1 -> JointTorqueDes_Nm/1

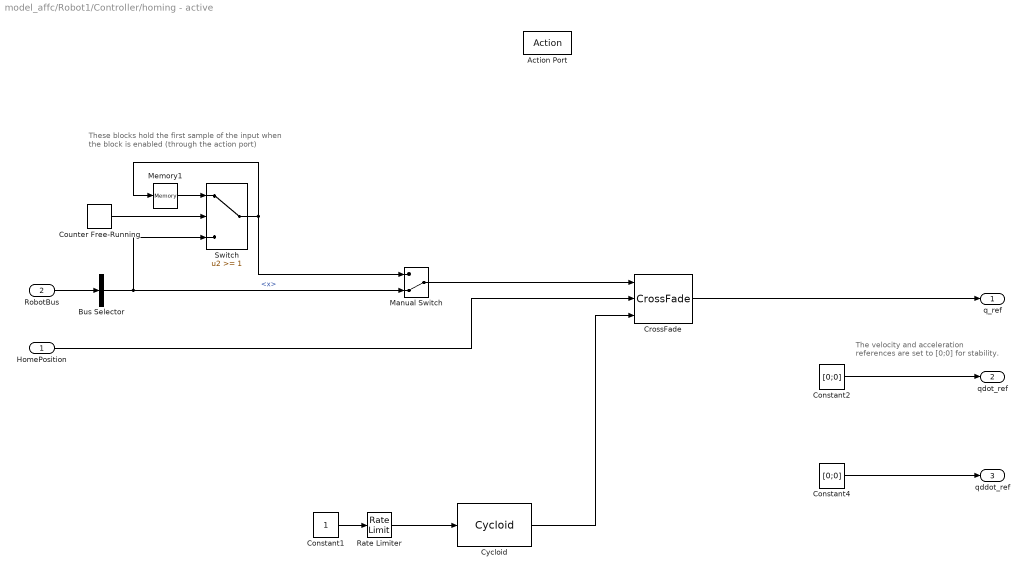
== system model_affc/Robot1/Controller/homing - active ==
  note: These blocks hold the first sample of the input
      | when the block is enabled (through the action port)
  note: The velocity and acceleration references are set to [0;0] for stability.
  HomePosition : Inport
  RobotBus : Inport  Port=2
  Action Port : ActionPort  InitializeStates=reset  ActionType=case
  Bus Selector : BusSelector  OutputSignals=xOpSpace.x
  Constant1 : Constant
  Constant2 : Constant  Value=[0;0]
  Constant4 : Constant  Value=[0;0]
  Counter Free-Running : simulink/Sources/Counter Free-Running  NumBits=32  tsamp=-1
  CrossFade : VariousBlocksLibrary/Various/CrossFade
  Cycloid : VariousBlocksLibrary/Various/Cycloid
  Manual Switch : ManualSwitch  CurrentSetting=0
  Memory1 : Memory
  Rate Limiter : RateLimiter  RisingSlewLimit=0.2  FallingSlewLimit=-0.2  SampleTimeMode=inherited
  Switch : Switch  Threshold=1
  q_ref : Outport  OutputWhenDisabled=reset  InitialOutput=[0;0]
  qdot_ref : Outport  Port=2  OutputWhenDisabled=reset  InitialOutput=[0;0]
  qddot_ref : Outport  Port=3  OutputWhenDisabled=reset  InitialOutput=[0;0]
  wires:
  Constant2/1 -> qdot_ref/1
  Bus Selector/1 -> Manual Switch/2, Switch/3  "<x>"
  RobotBus/1 -> Bus Selector/1
  HomePosition/1 -> CrossFade/2
  Cycloid/1 -> CrossFade/3
  Rate Limiter/1 -> Cycloid/1
  Constant1/1 -> Rate Limiter/1
  Switch/1 -> Memory1/1, Manual Switch/1
  Counter Free-Running/1 -> Switch/2
  Memory1/1 -> Switch/1
  Manual Switch/1 -> CrossFade/1
  CrossFade/1 -> q_ref/1
  Constant4/1 -> qddot_ref/1

== system model_affc/Robot1/Controller/homing - done ==
  Action Port : ActionPort  ActionType=case
  Constant : Constant  Value=[0;0]
  JointTorqueDes_Nm : Outport  InitialOutput=[0;0]
  wires:
  Constant/1 -> JointTorqueDes_Nm/1

== system model_affc/Robot1/Controller/idle (no torque) ==
  Action Port : ActionPort  InitializeStates=reset  ActionType=case
  Constant3 : Constant  Value=[0;0]
  JointTorqueDes_Nm : Outport  InitialOutput=[0;0]
  wires:
  Constant3/1 -> JointTorqueDes_Nm/1

== system model_affc/Robot1/Controller/run ==
  q_ref_in : Inport
  qdot_ref_in : Inport  Port=2
  qddot_ref_in : Inport  Port=3
  Action Port : ActionPort  InitializeStates=reset  ActionType=case
  q_ref : Outport  OutputWhenDisabled=reset  InitialOutput=[0;0]
  qdot_ref : Outport  Port=2  OutputWhenDisabled=reset  InitialOutput=[0;0]
  qddot_ref : Outport  Port=3  OutputWhenDisabled=reset  InitialOutput=[0;0]
  wires:
  qdot_ref_in/1 -> qdot_ref/1
  qddot_ref_in/1 -> qddot_ref/1
  q_ref_in/1 -> q_ref/1

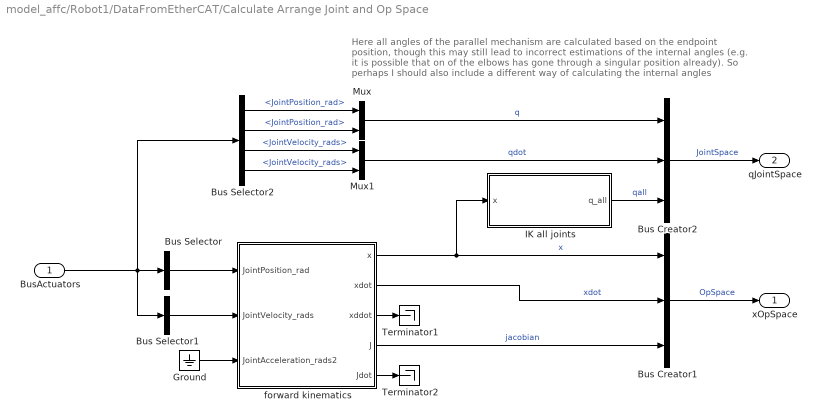
== system model_affc/Robot1/DataFromEtherCAT/Calculate Arrange Joint and Op Space ==
  note: Here all angles of the parallel mechanism are calculated
      | based on the endpoint position, though this may still lead to incorrect
      | estimations of the internal angles (e.g. it is possible that on of the elbows
      | has gone through a singular position already). So perhaps I should also include
      | a different way of calculating the internal angles
  BusActuators : Inport
  Bus Creator1 : BusCreator  Inputs=3
  Bus Creator2 : BusCreator  Inputs=3
  Bus Selector : BusSelector  OutputSignals=BusActuator1.JointPosition_rad,BusActuator2.JointPosition_rad  OutputAsBus=on
  Bus Selector1 : BusSelector  OutputSignals=BusActuator1.JointVelocity_rads,BusActuator2.JointVelocity_rads  OutputAsBus=on
  Bus Selector2 : BusSelector  OutputSignals=BusActuator1.JointPosition_rad,BusActuator2.JointPosition_rad,BusActuator1.JointVelocity_rads,BusActuator2.JointVelocity_rads
  Ground : Ground
  IK all joints : MATLAB Function  TreatAsAtomicUnit=on
  Mux : Mux  Inputs=2
  Mux1 : Mux  Inputs=2
  Terminator1 : Terminator
  Terminator2 : Terminator
  forward kinematics : Subsystem
  xOpSpace : Outport
  qJointSpace : Outport  Port=2
  wires:
  forward kinematics/5(Jdot) -> Terminator2/1
  forward kinematics/3(xddot) -> Terminator1/1
  forward kinematics/2(xdot) -> Bus Creator1/2  "xdot"
  Bus Selector/1 -> forward kinematics/1(JointPosition_rad)
  forward kinematics/1(x) -> IK all joints/1(x), Bus Creator1/1  "x"
  Bus Creator1/1 -> xOpSpace/1  "OpSpace"
  forward kinematics/4(J) -> Bus Creator1/3  "jacobian"
  Bus Selector1/1 -> forward kinematics/2(JointVelocity_rads)
  Ground/1 -> forward kinematics/3(JointAcceleration_rads2)
  Bus Creator2/1 -> qJointSpace/1  "JointSpace"
  BusActuators/1 -> Bus Selector1/1, Bus Selector2/1, Bus Selector/1
  Mux/1 -> Bus Creator2/1  "q"
  Bus Selector2/1 -> Mux/1  "<JointPosition_rad>"
  Bus Selector2/2 -> Mux/2  "<JointPosition_rad>"
  Bus Selector2/3 -> Mux1/1  "<JointVelocity_rads>"
  Bus Selector2/4 -> Mux1/2  "<JointVelocity_rads>"
  Mux1/1 -> Bus Creator2/2  "qdot"
  IK all joints/1(q_all) -> Bus Creator2/3  "qall"

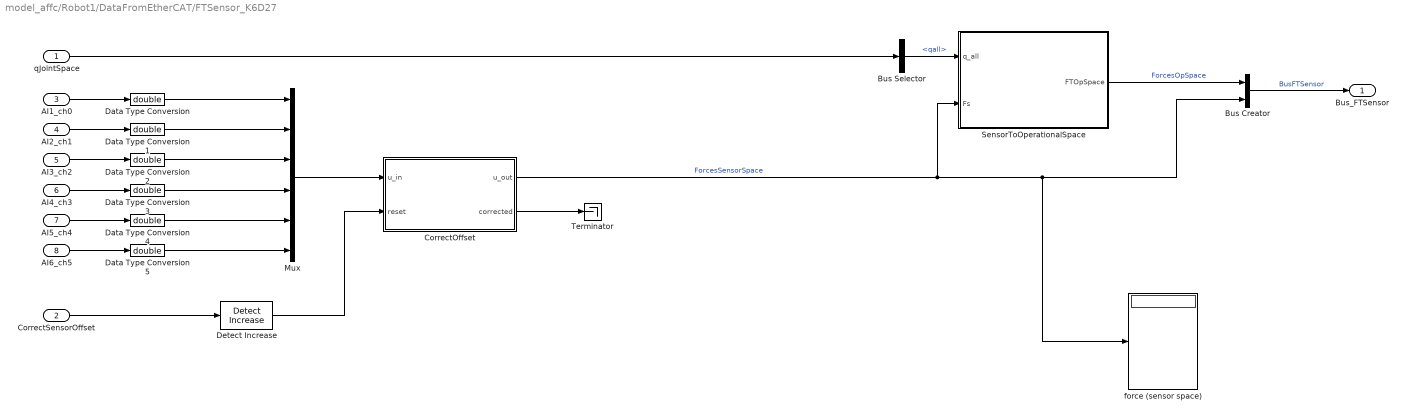
== system model_affc/Robot1/DataFromEtherCAT/FTSensor_K6D27 ==
  qJointSpace : Inport
  CorrectSensorOffset : Inport  Port=2
  AI1_ch0 : Inport  Port=3
  AI2_ch1 : Inport  Port=4
  AI3_ch2 : Inport  Port=5
  AI4_ch3 : Inport  Port=6
  AI5_ch4 : Inport  Port=7
  AI6_ch5 : Inport  Port=8
  Bus Creator : BusCreator  Inputs=2
  Bus Selector : BusSelector  OutputSignals=qall
  CorrectOffset : MATLAB Function  TreatAsAtomicUnit=on
  Data Type Conversion{,1..5} (6 alike) : DataTypeConversion  OutDataTypeStr=double
  Detect Increase : simulink/Logic and Bit Operations/Detect Increase  vinit=0.0  InputProcessing=Inherited  OutDataTypeStr=boolean
  Mux : Mux  Inputs=6
  SensorToOperationalSpace : MATLAB Function  TreatAsAtomicUnit=on
  Terminator : Terminator
  force (sensor space) : Display
  Bus_FTSensor : Outport
  wires:
  qJointSpace/1 -> Bus Selector/1
  AI2_ch1/1 -> Data Type Conversion1/1
  AI1_ch0/1 -> Data Type Conversion/1
  Mux/1 -> CorrectOffset/1(u_in)
  CorrectSensorOffset/1 -> Detect Increase/1
  Detect Increase/1 -> CorrectOffset/2(reset)
  Bus Selector/1 -> SensorToOperationalSpace/1(q_all)  "<qall>"
  AI6_ch5/1 -> Data Type Conversion5/1
  AI5_ch4/1 -> Data Type Conversion4/1
  AI4_ch3/1 -> Data Type Conversion3/1
  AI3_ch2/1 -> Data Type Conversion2/1
  CorrectOffset/2(corrected) -> Terminator/1
  CorrectOffset/1(u_out) -> Bus Creator/2, force (sensor space)/1, SensorToOperationalSpace/2(Fs)  "ForcesSensorSpace"
  Data Type Conversion/1 -> Mux/1
  Data Type Conversion1/1 -> Mux/2
  Data Type Conversion2/1 -> Mux/3
  Data Type Conversion3/1 -> Mux/4
  Data Type Conversion4/1 -> Mux/5
  Data Type Conversion5/1 -> Mux/6
  SensorToOperationalSpace/1(FTOpSpace) -> Bus Creator/1  "ForcesOpSpace"
  Bus Creator/1 -> Bus_FTSensor/1  "BusFTSensor"

== system model_affc/Robot1/DataToEtherCAT/FTSensorError ==
  RobotBus : Inport
  AvoidAlgebraicLoop : Memory
  Bus Selector : BusSelector  OutputSignals=BusFTSensor.ForcesSensorSpace
  Constant : Constant  Value=RobotStruct.FTSensor.MaxAllowableForcesTorqueSensor
  CreateSingleErrorValue : LibraryFM/ToActuator1/DriveEnableLogic/CreateSingleErrorValue
  Detect Change : simulink/Logic and Bit Operations/Detect Change  vinit=0  InputProcessing=Inherited  OutDataTypeStr=boolean
  FTSensorLastError : Display
  LatchRising : LibraryFM/Utilities/LatchRising  ic=0
  MATLAB Function : MATLAB Function  TreatAsAtomicUnit=on
  ShowFTSensorErrorLatched : Display
  FTSensorError : Outport
  FTSensorErrorLatched : Outport  Port=2
  wires:
  Bus Selector/1 -> MATLAB Function/1(ForcesTorques)  "<ForcesSensorSpace>"
  RobotBus/1 -> Bus Selector/1
  Detect Change/1 -> LatchRising/Trigger
  AvoidAlgebraicLoop/1 -> FTSensorError/1, LatchRising/1, Detect Change/1
  LatchRising/1 -> FTSensorErrorLatched/1, ShowFTSensorErrorLatched/1
  CreateSingleErrorValue/1 -> AvoidAlgebraicLoop/1
  MATLAB Function/1(e) -> CreateSingleErrorValue/1, FTSensorLastError/1
  Constant/1 -> MATLAB Function/2(MaxForcesTorques)

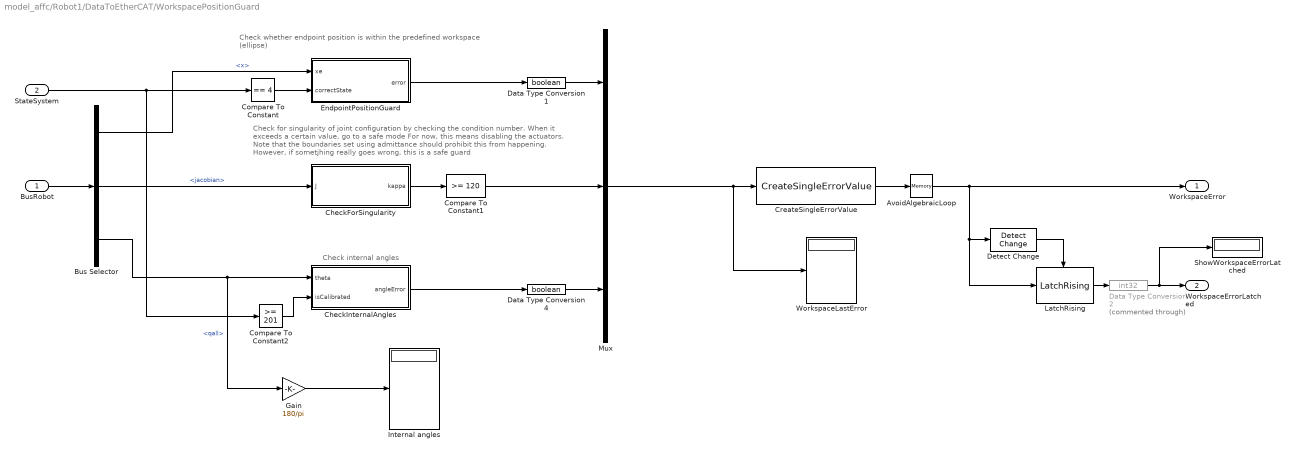
== system model_affc/Robot1/DataToEtherCAT/WorkspacePositionGuard ==
  note: Check internal angles
  note: Check whether endpoint position is within the predefined workspace
      | (ellipse)
  note: Check for singularity of joint configuration by checking
      | the condition number. When it exceeds a certain value, go to a safe mode
      | For now, this means disabling the actuators.
      | Note that the boundaries set using admittance should prohibit this from happening.
      | However, if sometjhing really goes wrong, this is a safe guard
  BusRobot : Inport
  StateSystem : Inport  Port=2
  AvoidAlgebraicLoop : Memory
  Bus Selector : BusSelector  OutputSignals=xOpSpace.x,xOpSpace.jacobian,qJointSpace.qall
  CheckForSingularity : MATLAB Function  TreatAsAtomicUnit=on
  CheckInternalAngles : MATLAB Function  TreatAsAtomicUnit=on
  Compare To Constant : simulink/Logic and Bit Operations/Compare To Constant  relop===  const=4  OutDataTypeStr=boolean
  Compare To Constant1 : simulink/Logic and Bit Operations/Compare To Constant  relop=>=  const=120  OutDataTypeStr=boolean
  Compare To Constant2 : simulink/Logic and Bit Operations/Compare To Constant  relop=>=  const=201  OutDataTypeStr=boolean
  CreateSingleErrorValue : LibraryFM/ToActuator1/DriveEnableLogic/CreateSingleErrorValue
  Data Type Conversion1 : DataTypeConversion  OutDataTypeStr=boolean
  Data Type Conversion2 : DataTypeConversion  Commented=through  OutDataTypeStr=int32
  Data Type Conversion4 : DataTypeConversion  OutDataTypeStr=boolean
  Detect Change : simulink/Logic and Bit Operations/Detect Change  vinit=0  InputProcessing=Inherited  OutDataTypeStr=boolean
  EndpointPositionGuard : MATLAB Function  TreatAsAtomicUnit=on
  Gain : Gain  Gain=180/pi
  Internal angles : Display
  LatchRising : LibraryFM/Utilities/LatchRising  ic=0
  Mux : Mux  Inputs=3
  ShowWorkspaceErrorLatched : Display
  WorkspaceLastError : Display
  WorkspaceError : Outport
  WorkspaceErrorLatched : Outport  Port=2
  wires:
  CheckForSingularity/1(kappa) -> Compare To Constant1/1
  Mux/1 -> CreateSingleErrorValue/1, WorkspaceLastError/1
  BusRobot/1 -> Bus Selector/1
  Bus Selector/1 -> EndpointPositionGuard/1(xe)  "<x>"
  Bus Selector/3 -> Gain/1, CheckInternalAngles/1(theta)  "<qall>"
  LatchRising/1 -> Data Type Conversion2/1
  EndpointPositionGuard/1(error) -> Data Type Conversion1/1
  CheckInternalAngles/1(angleError) -> Data Type Conversion4/1
  CreateSingleErrorValue/1 -> AvoidAlgebraicLoop/1
  Detect Change/1 -> LatchRising/Trigger
  AvoidAlgebraicLoop/1 -> LatchRising/1, Detect Change/1, WorkspaceError/1
  Compare To Constant/1 -> EndpointPositionGuard/2(correctState)
  Compare To Constant2/1 -> CheckInternalAngles/2(isCalibrated)
  Gain/1 -> Internal angles/1
  Bus Selector/2 -> CheckForSingularity/1(J)  "<jacobian>"
  StateSystem/1 -> Compare To Constant2/1, Compare To Constant/1
  Data Type Conversion2/1 -> ShowWorkspaceErrorLatched/1, WorkspaceErrorLatched/1
  Data Type Conversion1/1 -> Mux/1
  Compare To Constant1/1 -> Mux/2
  Data Type Conversion4/1 -> Mux/3

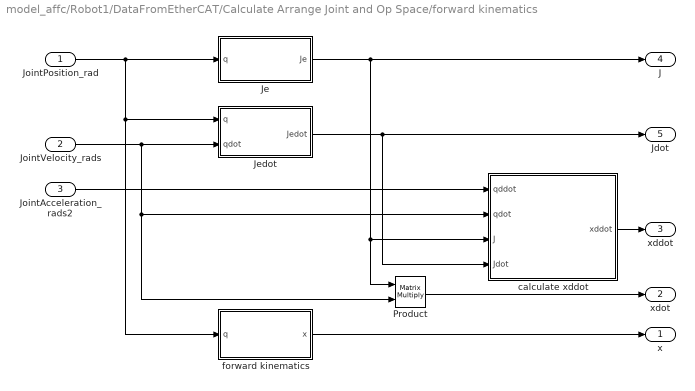
== system model_affc/Robot1/DataFromEtherCAT/Calculate Arrange Joint and Op Space/forward kinematics ==
  JointPosition_rad : Inport  PortDimensions=[2 1]
  JointVelocity_rads : Inport  Port=2  PortDimensions=[2 1]
  JointAcceleration_rads2 : Inport  Port=3  PortDimensions=[2 1]
  Je : MATLAB Function  TreatAsAtomicUnit=on
  Jedot : MATLAB Function  TreatAsAtomicUnit=on
  Product : Product  Multiplication=Matrix(*)
  calculate xddot : MATLAB Function  TreatAsAtomicUnit=on
  forward kinematics : MATLAB Function  TreatAsAtomicUnit=on
  x : Outport
  xdot : Outport  Port=2
  xddot : Outport  Port=3
  J : Outport  Port=4
  Jdot : Outport  Port=5
  wires:
  JointPosition_rad/1 -> forward kinematics/1(q), Jedot/1(q), Je/1(q)
  Je/1(Je) -> calculate xddot/3(J), Product/1, J/1
  JointVelocity_rads/1 -> calculate xddot/2(qdot), Product/2, Jedot/2(qdot)
  Jedot/1(Jedot) -> calculate xddot/4(Jdot), Jdot/1
  Product/1 -> xdot/1
  forward kinematics/1(x) -> x/1
  calculate xddot/1(xddot) -> xddot/1
  JointAcceleration_rads2/1 -> calculate xddot/1(qddot)

== matlab function model_affc/Robot1/DataToEtherCAT/FTSensorError/MATLAB Function ==
  data: ForcesTorques input; e output; MaxForcesTorques input
function e = fcn(ForcesTorques, MaxForcesTorques)

% throw error when any of the forces/torques go over a max allowable value
if any(abs(ForcesTorques) > MaxForcesTorques) 
    e = 1;
else
    e = 0;
end

== matlab function model_affc/Robot1/DataFromEtherCAT/Calculate Arrange Joint and Op Space/forward kinematics/forward kinematics ==
  data: q input; x output size=[2 1]; Lf parameter; Lu parameter; Lb parameter
function x = FK(q, Lf, Lu, Lb)
%#codegen

% Calculate the endpoint position (forward kinematics)
% Note that the function func_eq_FK needs to be in the libraries/kinematis_functions folder


x = func_eq_FK(q(1),q(2),Lf,Lu,Lb);

== matlab function model_affc/Robot1/Controller/inverse kinematics1 ==
  data: x input; q output size=[2 1]; Lf parameter; Lu parameter; Lb parameter
function q  = IK(x,Lf,Lu,Lb)
%#codegen

% inverse dynamics
q = func_eq_IK(x(1),x(2),Lf,Lu,Lb);

== matlab function model_affc/Haptics/Hypotrochoid trajectory for AFFC/hypotrochoidal trajectory ==
  data: t input; p output; v output; a output; T input; n input; hstart input; hend input; wstart input; wend input
function [p,v,a] = fcn(t,T,n,hstart,hend,wstart,wend)
%#codegen

p = func_p_hypothrochoid(t,T,n,hstart,hend,wstart,wend);
v = func_v_hypothrochoid(t,T,n,hstart,hend,wstart,wend);
a = func_a_hypothrochoid(t,T,n,hstart,hend,wstart,wend);

== matlab function model_affc/Robot1/DataFromEtherCAT/Calculate Arrange Joint and Op Space/forward kinematics/Je ==
  data: q input; Je output size=[2 2]; Lf parameter; Lu parameter; Lb parameter
function Je = Je( q, Lf, Lu, Lb)
%#codegen

% Calculate the Jacobian for this particular device configuration.
% Note that the function func_eq_Je needs to be in the libraries/kinematis_functions folder

% jacobians
Je = func_eq_Je(q(1),q(2),Lf,Lu,Lb);

== matlab function model_affc/Robot1/DataFromEtherCAT/Calculate Arrange Joint and Op Space/forward kinematics/Jedot ==
  data: q input; qdot input; Jedot output size=[2 2]; Lf parameter; Lu parameter; Lb parameter
function Jedot = Jedot( q, qdot, Lf, Lu, Lb)
%#codegen

% Calculate the time derivative of the Jacobian for this particular device configuration.
% Note that the function func_eq_Je needs to be in the libraries/kinematis_functions folder


% jacobians
Jedot = func_eq_Jedot(q(1),q(2),qdot(1),qdot(2),Lf,Lu,Lb);

== matlab function model_affc/Robot1/DataFromEtherCAT/FTSensor_K6D27/CorrectOffset ==
  data: u_in input; u_out output; reset input; corrected output
function [u_out,corrected] = CorrectOffset(u_in,reset)
%#codegen

persistent data_ offset_ counter_ corrected_;
N = 1000;

% initialize
if isempty(data_)
    data_ = zeros(size(u_in,1), N);
    offset_ = zeros(size(u_in));
    counter_ = 1;
    corrected_ = 0;
end

if (counter_ <= N)
    data_(:,counter_) = u_in;
end

counter_ = counter_ + 1;
if reset
    counter_ = 1;
end

% calculate mean
if counter_ == N
    corrected_ = 1;
    offset_ = mean(data_,2);
end

corrected = corrected_;
u_out = u_in - offset_;

== matlab function model_affc/Robot1/DataFromEtherCAT/Calculate Arrange Joint and Op Space/IK all joints ==
  data: x input; q_all output; Lf parameter; Lu parameter; Lb parameter
function q_all = IK_all(x,Lf,Lu,Lb)
%#codegen

if (x(2) >= 0.07)
    q_all = func_eqs_IK_all(x(1),x(2),Lf,Lu,Lb);
else
    x = [0;0.07];
    q_all = func_eqs_IK_all(x(1),x(2),Lf,Lu,Lb);
end

== matlab function model_affc/Robot1/DataFromEtherCAT/Calculate Arrange Joint and Op Space/forward kinematics/calculate xddot ==
  data: qddot input; qdot input size=[2 1]; J input; xddot output size=[2 1]; Jdot input
function xddot = calc_xddot(qddot, qdot, J, Jdot)
%#codegen

xddot = J*qddot + Jdot*qdot;

== matlab function model_affc/Robot1/Controller/inverse kinematics ==
  data: x input; xdot input; xddot input; q output size=[2 1]; Lf parameter; Lu parameter; Lb parameter; qdot output; qddot output
function [q,qdot,qddot] = IK(x,xdot,xddot,Lf,Lu,Lb)
%#codegen

% inverse dynamics
q = func_eq_IK(x(1),x(2),Lf,Lu,Lb);

% jacobians
Je = func_eq_Je(q(1),q(2),Lf,Lu,Lb);

% calculate qdot
qdot = pinv(Je)*xdot;

% calculate qddot
Jedot = func_eq_Jedot(q(1),q(2),qdot(1),qdot(2),Lf,Lu,Lb);
qddot = pinv(Je)*(xddot-Jedot*qdot);

== matlab function model_affc/Robot1/DataFromEtherCAT/FTSensor_K6D27/SensorToOperationalSpace ==
  data: q_all input; Fs input; FTOpSpace output
function FTOpSpace = ForceSensorToOperationalSpace(q_all,Fs)
%#codegen

% select correct angles. Note! During assembly we weren't very consistent
% to which forearm the sensor is fixed. For FM1 (green), the sensor is
% attached to arm 2, hence the rotation matrics are made using angles
% theta1 and theta2
% rotation matrices (I derived them from actuator 1 to endpoint, but
% transformation is other way around (i.e. inverse). Since inverse calculation 
% could take some time, Could be done by
% negating the angles instead of inverse of matrix.
q1 = q_all(1);
q2 = (pi-q_all(2)); % pi-theta2 since theta2 is the internal angle of this joint

R = [-cos(q1+q2) sin(q1+q2);-sin(q1+q2) -cos(q1+q2)];

% transform force
FTOpSpace = R*Fs(1:2);

== matlab function model_affc/Robot1/DataToEtherCAT/WorkspacePositionGuard/CheckForSingularity ==
  data: J input; kappa output
function kappa = conditionnumber(J)
%#codegen

kappa = norm(pinv(J))*norm(J);

== matlab function model_affc/Robot1/DataToEtherCAT/WorkspacePositionGuard/CheckInternalAngles ==
  data: theta input; angleError output; isCalibrated input
function angleError = checkInternalErrors(theta,isCalibrated)
%#codegen

angleError = 0;

if isCalibrated
    % check whether theta2 or theta4 are smaller than 0.95*pi. If larger, throw
    % error
    if any(theta([2 4]) >= 0.95*pi)
        angleError = 1;
    end
end

== matlab function model_affc/Robot1/DataToEtherCAT/WorkspacePositionGuard/EndpointPositionGuard ==
  data: xe input; error output; correctState input
function error = fcn(xe, correctState)
%#codegen


error = 0;

% only check workspace boundaries after homing state is done
if ~correctState 
    return; 
end

% x0 = 0;
% y0 = 0.2354;
% a = 0.11;
% b = 0.08;

% workspace (see design document)
x0 = 0;
y0 = 0.25024;
a = 0.1746;
b = 0.13;%0.1048;

% check if endpoint is outside a predefined ellipse
x = xe(1);
y = xe(2);

% workspace is defined as an ellipse
e = (x-x0)^2 / a^2 + (y-y0)^2 / b^2;

% if is larger than 1, the endpoint is outside the workspace
if e > 1
    error = 1;
end
